simulink model "Rad_2node"  (R2018b)
settings: Solver=FixedStepAuto  StartTime=0.0  StopTime=100000  FixedStep=5  RelTol=1e-3
undefined symbols (not defined in the file or in its folder): DiscIntNeverNeededParam
settings Model: Creator=cpp14rcj  LastModifiedBy=cpp14rcj

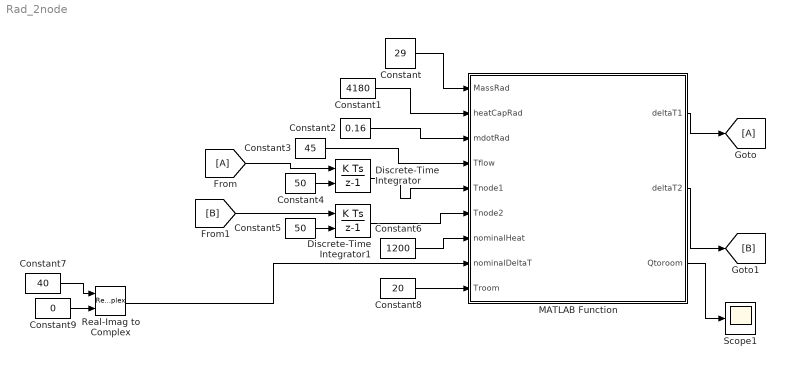
== system Rad_2node ==
  Constant : Constant  Value=29
  Constant1 : Constant  Value=4180
  Constant2 : Constant  Value=0.16
  Constant3 : Constant  Value=45
  Constant4 : Constant  Value=50
  Constant5 : Constant  Value=50
  Constant6 : Constant  Value=1200
  Constant7 : Constant  Value=40
  Constant8 : Constant  Value=20
  Constant9 : Constant  Value=0
  Discrete-Time Integrator : DiscreteIntegrator  InitialConditionSource=external  SampleTime=-1  ICPrevOutput=DiscIntNeverNeededParam  ICPrevScaledInput=DiscIntNeverNeededParam
  Discrete-Time Integrator1 : DiscreteIntegrator  InitialConditionSource=external  SampleTime=-1  ICPrevOutput=DiscIntNeverNeededParam  ICPrevScaledInput=DiscIntNeverNeededParam
  MATLAB Function : MATLAB Function  TreatAsAtomicUnit=on
  Real-Imag to Complex : RealImagToComplex
  Scope1 : Scope
  wires:
  Constant/1 -> MATLAB Function/1(MassRad)
  Constant1/1 -> MATLAB Function/2(heatCapRad)
  Constant2/1 -> MATLAB Function/3(mdotRad)
  Constant3/1 -> MATLAB Function/4(Tflow)
  Constant4/1 -> Discrete-Time Integrator/2
  Discrete-Time Integrator/1 -> MATLAB Function/5(Tnode1)
  Constant5/1 -> Discrete-Time Integrator1/2
  Discrete-Time Integrator1/1 -> MATLAB Function/6(Tnode2)
  [A] -> Discrete-Time Integrator/1
  MATLAB Function/1(deltaT1) -> [A]
  [B] -> Discrete-Time Integrator1/1
  MATLAB Function/2(deltaT2) -> [B]
  Constant6/1 -> MATLAB Function/7(nominalHeat)
  Constant7/1 -> Real-Imag to Complex/1
  Constant8/1 -> MATLAB Function/9(Troom)
  Constant9/1 -> Real-Imag to Complex/2
  Real-Imag to Complex/1 -> MATLAB Function/8(nominalDeltaT)
  MATLAB Function/3(Qtoroom) -> Scope1/1

== matlab function Rad_2node/MATLAB Function ==
  data: MassRad input; heatCapRad input; mdotRad input; Tflow input; Tnode1 input; Tnode2 input; deltaT1 output; deltaT2 output; nominalHeat input; nominalDeltaT input; Troom input; Qtoroom output
function [deltaT1,deltaT2,Qtoroom]=fcn(MassRad,heatCapRad, mdotRad, Tflow,Tnode1,Tnode2,nominalHeat,nominalDeltaT,Troom)


if  Tnode1 == Tnode2 || Tnode1 <= Troom || Tnode2 <= Troom %if lmtd methodnis problemtatic, use arithmetic method
    radiatorHeatOut=sign(((Tnode1+Tnode2) /2)-Troom)*abs((nominalHeat)*((((Tnode1+Tnode2) /2)-Troom)/nominalDeltaT)^1.3);
deltaT1=(mdotRad*4180*(Tflow-Tnode1))/((heatCapRad*MassRad)/2);
deltaT2=(mdotRad*4180*(Tnode1-Tnode2)-radiatorHeatOut)/((heatCapRad*MassRad)/2);

else 
  
   radiatorHeatOut=(nominalHeat/nominalDeltaT^1.3)*((Tnode1-Tnode2)/log((Tnode1-Troom)/(Tnode2-Troom)))^1.3;
   radiatorHeatOut=real(radiatorHeatOut);
deltaT1=(mdotRad*4180*(Tflow-Tnode1))/((heatCapRad*MassRad)/2);
deltaT2=(mdotRad*4180*(Tnode1-Tnode2)-radiatorHeatOut)/((heatCapRad*MassRad)/2);

   deltaT1=real(deltaT1);
   deltaT2=real(deltaT2);
    

end

Qtoroom=real(radiatorHeatOut);
